simulink model "mac_simulink"  (R2024b)
settings: Solver=VariableStepAuto  StartTime=0.0  StopTime=39  RelTol=1e-3
settings Model: Creator=aherrman  LastModifiedBy=aherrman

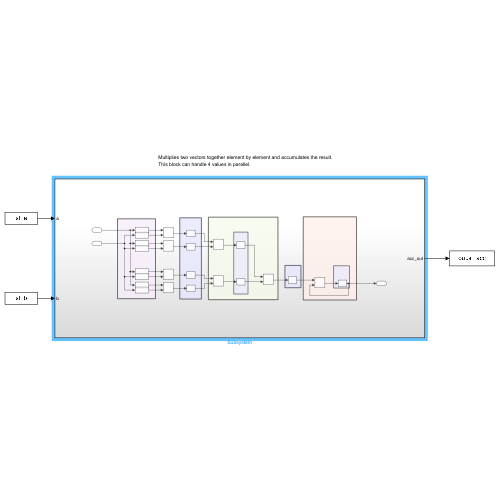
[thumbnail: Simulink's stored preview of the top-level diagram]
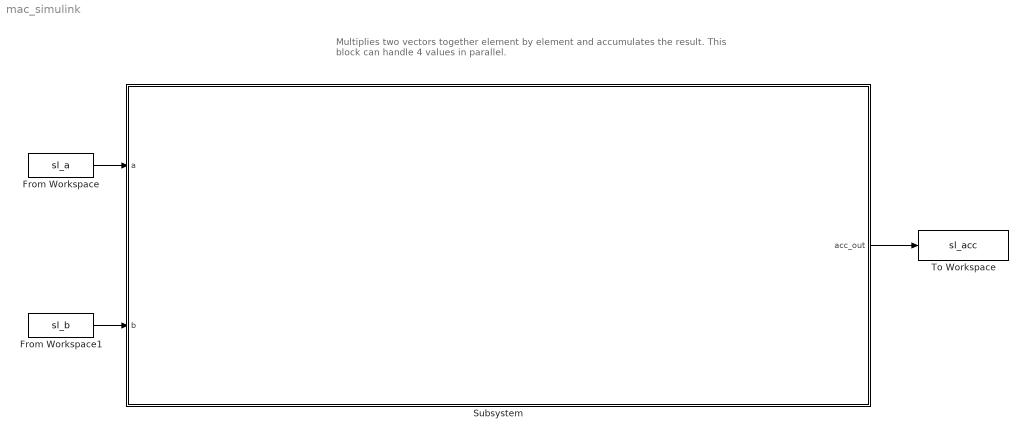
== system mac_simulink ==
  note: Multiplies two vectors together element by element and accumulates the result.
      | This block can handle 4 values in parallel.
  From Workspace : FromWorkspace  VariableName=sl_a  SampleTime=1  OutputAfterFinalValue=Setting to zero
  From Workspace1 : FromWorkspace  VariableName=sl_b  SampleTime=1  OutputAfterFinalValue=Setting to zero
  Subsystem : Subsystem
  To Workspace : ToWorkspace  VariableName=sl_acc  SaveFormat=Timeseries  SampleTime=-1
  wires:
  From Workspace/1 -> Subsystem/1(a)
  From Workspace1/1 -> Subsystem/2(b)
  Subsystem/1(acc_out) -> To Workspace/1

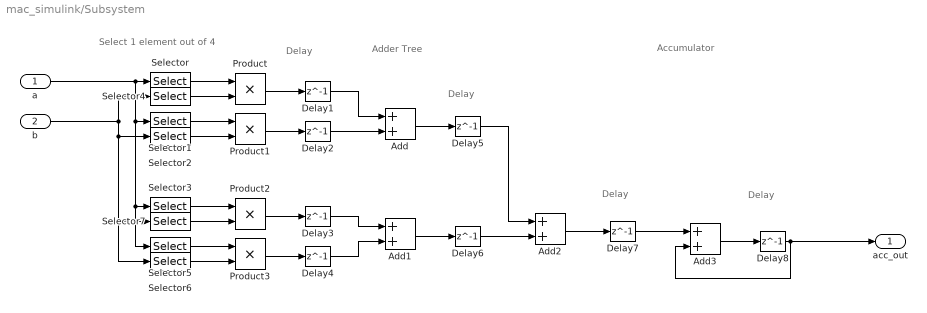
== system mac_simulink/Subsystem ==
  note: Accumulator
  note: Adder Tree
  note: Select 1 element
      | out of 4
  note: Delay
  note: Delay
  note: Delay
  note: Delay
  a : Inport
  b : Inport  Port=2
  Add{,1..3} (4 alike) : Sum
  Delay{1..8} (8 alike) : Delay  DelayLength=1
  Product{,1..3} (4 alike) : Product
  Selector : Selector  IndexMode=Zero-based  InputPortWidth=4  IndexOptions=Index vector (dialog)  Indices=[0]  OutputSizes=1
  Selector1 : Selector  IndexMode=Zero-based  InputPortWidth=4  IndexOptions=Index vector (dialog)  Indices=[1]  OutputSizes=1
  Selector2 : Selector  IndexMode=Zero-based  InputPortWidth=4  IndexOptions=Index vector (dialog)  Indices=[1]  OutputSizes=1
  Selector3 : Selector  IndexMode=Zero-based  InputPortWidth=4  IndexOptions=Index vector (dialog)  Indices=[2]  OutputSizes=1
  Selector4 : Selector  IndexMode=Zero-based  InputPortWidth=4  IndexOptions=Index vector (dialog)  Indices=[0]  OutputSizes=1
  Selector5 : Selector  IndexMode=Zero-based  InputPortWidth=4  IndexOptions=Index vector (dialog)  Indices=[3]  OutputSizes=1
  Selector6 : Selector  IndexMode=Zero-based  InputPortWidth=4  IndexOptions=Index vector (dialog)  Indices=[3]  OutputSizes=1
  Selector7 : Selector  IndexMode=Zero-based  InputPortWidth=4  IndexOptions=Index vector (dialog)  Indices=[2]  OutputSizes=1
  acc_out : Outport
  wires:
  Selector5/1 -> Product3/1
  Delay7/1 -> Add3/1
  Delay3/1 -> Add1/1
  b/1 -> Selector2/1, Selector7/1, Selector6/1, Selector4/1
  Add/1 -> Delay5/1
  Delay8/1 -> acc_out/1, Add3/2
  a/1 -> Selector5/1, Selector3/1, Selector1/1, Selector/1
  Delay5/1 -> Add2/1
  Selector/1 -> Product/1
  Product2/1 -> Delay3/1
  Selector2/1 -> Product1/2
  Add1/1 -> Delay6/1
  Delay4/1 -> Add1/2
  Delay6/1 -> Add2/2
  Add3/1 -> Delay8/1
  Delay2/1 -> Add/2
  Product3/1 -> Delay4/1
  Selector1/1 -> Product1/1
  Product1/1 -> Delay2/1
  Add2/1 -> Delay7/1
  Product/1 -> Delay1/1
  Selector7/1 -> Product2/2
  Selector6/1 -> Product3/2
  Delay1/1 -> Add/1
  Selector4/1 -> Product/2
  Selector3/1 -> Product2/1
